simulink model "Double_track_model"  (R2025b)
settings: Solver=VariableStepAuto  StartTime=0.0  StopTime=100  MaxStep=0.001  RelTol=1e-4
model workspace (MAT data in the model file):
  A = 1
  C1 = 1.2801
  C2 = 23.99
  C3 = 0.52
  Cd = 0.01
  Croll = 0.015
  Hcg = 0.25
  Iw = 0.65
  Izz = 100
  L = 1.535
  Lf = 0.78285
  Lr = 0.75215
  M = 270
  Rw = 0.228
  b = 0.1
  rho = 1.25
  tf = 1.24
  tr = 1.24
libraries: simulink x1
settings Model: SnapshotBufferSize=1000  SnapshotInterval=1  Creator=vishal bhujbal  LastModifiedBy=vishal bhujbal
settings DebuggingCC: AlgebraicLoopMsg=none

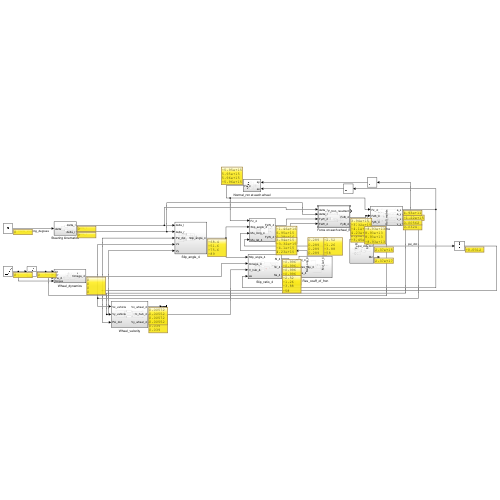
[thumbnail: Simulink's stored preview of the top-level diagram]
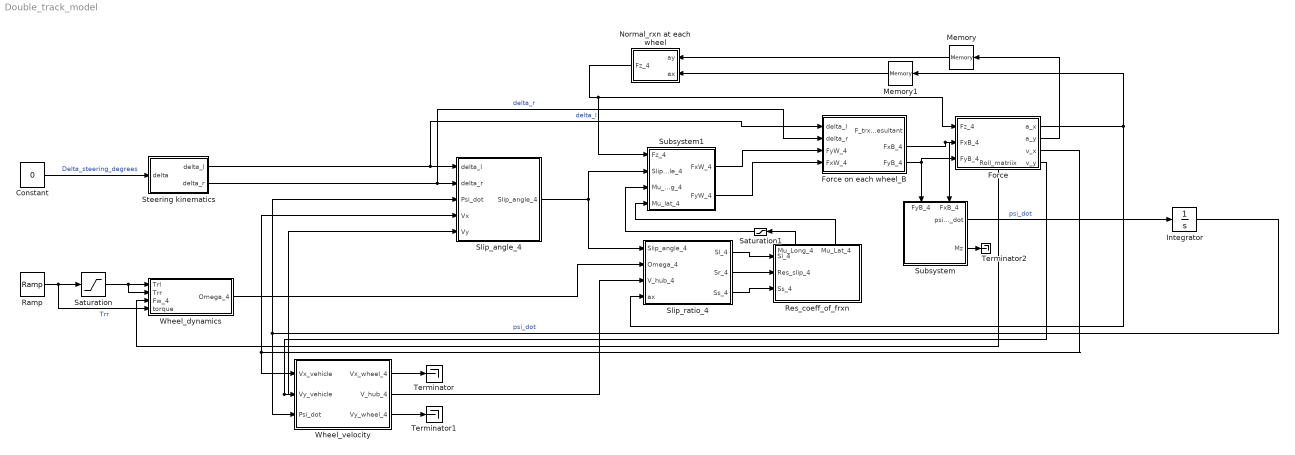
== system Double_track_model ==
  Constant : Constant  Value=0
  "Force " : Subsystem
      settings: PortSchema="{\"entries\":[{\"content\":{\"sides\":[{\"content\":{\"connectorIds\":[\"In1\",\"In2\",\"In3\"]},\"type\":\"ConnectorPlacement.EquallySpacedRectSide\",\"uuid\":\"d5a684a3-405b-4555-a50f-188f2a4da8d7\"},{\"content\":{\"connectorIds\":[\"Out1\",\"Out2\",\"Out3\",\"Out4\"],\"side\":\"RIGHT\"},\"type\":\"ConnectorPlacement.EquallySpacedRectSide\",\"uuid\":\"542d621c-7925-49ff-9525-88ce37fba4f5\"},{\"content\":{\"side\":\"TOP\"},\"type\":\"ConnectorPlacement.EquallySpacedRectSide\",\"uuid\":\"43f45826-7af5-4baa-927c-30d7ca0ba12e\"},{\"content\":{\"connectorIds\":[\"Out5\"],\"side\":\"BOTTOM\"},\"type\":\"ConnectorPlacement.EquallySpacedRectSide\",\"uuid\":\"968878bb-8701-45ce-acde-54180892fdcf\"}]},\"type\":\"ConnectorPlacement.EquallySpacedConnector\",\"uuid\":\"207dd83c-3604-4905-a41a-a8d49a457a53\"}],\"packageUris\":[\"http://schema.mathworks.com/mf0/Connector/R2020b\"],\"version\":\"1.0\"}"
  Force on each wheel_B : Subsystem
  Integrator : Integrator  InitialCondition=0.0001  ZeroCross=off
  Memory : Memory
  Memory1 : Memory
  Normal_rxn at each wheel : Subsystem
  Ramp : simulink/Sources/Ramp  slope=0  start=2  InitialOutput=0
  Res_coeff_of_frxn : Subsystem
      settings: PortSchema="{\"entries\":[{\"content\":{\"sides\":[{\"content\":{\"connectorIds\":[\"In1\",\"In2\",\"In3\"]},\"type\":\"ConnectorPlacement.EquallySpacedRectSide\",\"uuid\":\"69ce259e-3e29-48f3-954d-87ca310c7402\"},{\"content\":{\"side\":\"RIGHT\"},\"type\":\"ConnectorPlacement.EquallySpacedRectSide\",\"uuid\":\"84bf132b-ee57-474e-86e9-ab37d396531c\"},{\"content\":{\"connectorIds\":[\"Out1\",\"Out2\"],\"side\":\"TOP\"},\"type\":\"ConnectorPlacement.EquallySpacedRectSide\",\"uuid\":\"0b052469-b674-480c-8987-c0791ceb77cf\"}]},\"type\":\"ConnectorPlacement.EquallySpacedConnector\",\"uuid\":\"c5b7a706-d352-49d6-8b51-876ad1d5647c\"}],\"packageUris\":[\"http://schema.mathworks.com/mf0/Connector/R2020b\"],\"version\":\"1.0\"}"
  Saturation : Saturate  UpperLimit=29.1  LowerLimit=0
  Saturation1 : Saturate  UpperLimit=10  LowerLimit=-10
  Slip_angle_4 : Subsystem
  Slip_ratio_4 : Subsystem
  Steering kinematics : Subsystem
  Subsystem : Subsystem
      settings: PortSchema="{\"entries\":[{\"content\":{\"sides\":[{\"content\":{},\"type\":\"ConnectorPlacement.EquallySpacedRectSide\",\"uuid\":\"c1ec9233-0278-4624-8e9f-6381d2d56a9b\"},{\"content\":{\"connectorIds\":[\"Out1\",\"Out2\"],\"side\":\"RIGHT\"},\"type\":\"ConnectorPlacement.EquallySpacedRectSide\",\"uuid\":\"2db34302-ad88-4699-a49a-fe80526a01d5\"},{\"content\":{\"connectorIds\":[\"In1\",\"In2\"],\"side\":\"TOP\"},\"type\":\"ConnectorPlacement.EquallySpacedRectSide\",\"uuid\":\"531e9130-76c1-4daf-8db4-ad065a2e7511\"}]},\"type\":\"ConnectorPlacement.EquallySpacedConnector\",\"uuid\":\"470261c8-cc96-4ff8-80fc-dd2fad166e9a\"}],\"packageUris\":[\"http://schema.mathworks.com/mf0/Connector/R2020b\"],\"version\":\"1.0\"}"
  Subsystem1 : Subsystem
  Terminator : Terminator
  Terminator1 : Terminator
  Terminator2 : Terminator
  Wheel_dynamics : Subsystem
  Wheel_velocity : Subsystem
  wires:
  Steering kinematics/1(delta_l) -> Force on each wheel_B/1(delta_l), Slip_angle_4/1(delta_l)  "delta_l"
  Steering kinematics/2(delta_r) -> Force on each wheel_B/2(delta_r), Slip_angle_4/2(delta_r)  "delta_r"
  Constant/1 -> Steering kinematics/1(delta)  "Delta_steering_degrees"
  Wheel_dynamics/1(Omega_4) -> Slip_ratio_4/2(Omega_4)
  Slip_angle_4/1(Slip_angle_4) -> Subsystem1/2(Slip_angle_4), Slip_ratio_4/1(Slip_angle_4)
  Slip_ratio_4/2(Sr_4) -> Res_coeff_of_frxn/2(Res_slip_4)
  Slip_ratio_4/1(Sl_4) -> Res_coeff_of_frxn/1(Sl_4)
  Slip_ratio_4/3(Ss_4) -> Res_coeff_of_frxn/3(Ss_4)
  Normal_rxn at each wheel/1(Fz_4) -> Subsystem1/1(Fz_4), "Force "/1(Fz_4)
  Ramp/1 -> Wheel_dynamics/4(torque), Saturation/1  "Trr"
  Force on each wheel_B/2(FxB_4) -> Subsystem/2(FxB_4), "Force "/2(FxB_4)
  Force on each wheel_B/3(FyB_4) -> "Force "/3(FyB_4), Subsystem/1(FyB_4)
  "Force "/5(Roll_matriix) -> Wheel_dynamics/3(Fw_4)
  Subsystem/1(psi_dot_dot) -> Integrator/1  "psi_dot"
  Saturation/1 -> Wheel_dynamics/2(Trr), Wheel_dynamics/1(Trl)
  Wheel_velocity/3(Vy_wheel_4) -> Terminator1/1
  Wheel_velocity/1(Vx_wheel_4) -> Terminator/1
  Res_coeff_of_frxn/1(Mu_Long_4) -> Saturation1/1
  Res_coeff_of_frxn/2(Mu_Lat_4) -> Subsystem1/4(Mu_lat_4)
  Subsystem1/1(FxW_4) -> Force on each wheel_B/3(FyW_4)
  Subsystem1/2(FyW_4) -> Force on each wheel_B/4(FxW_4)
  "Force "/1(a_x) -> Memory1/1, Slip_ratio_4/4(ax)
  "Force "/2(a_y) -> Memory/1
  Subsystem/2(Mz) -> Terminator2/1
  Integrator/1 -> Wheel_velocity/3(Psi_dot), Slip_angle_4/3(Psi_dot)  "psi_dot"
  Saturation1/1 -> Subsystem1/3(Mu_long_4)
  Memory/1 -> Normal_rxn at each wheel/1(ay)
  Memory1/1 -> Normal_rxn at each wheel/2(ax)
  "Force "/3(v_x) -> Wheel_velocity/1(Vx_vehicle), Slip_angle_4/4(Vx)
  "Force "/4(v_y) -> Slip_angle_4/5(Vy), Wheel_velocity/2(Vy_vehicle)
  Wheel_velocity/2(V_hub_4) -> Slip_ratio_4/3(V_hub_4)

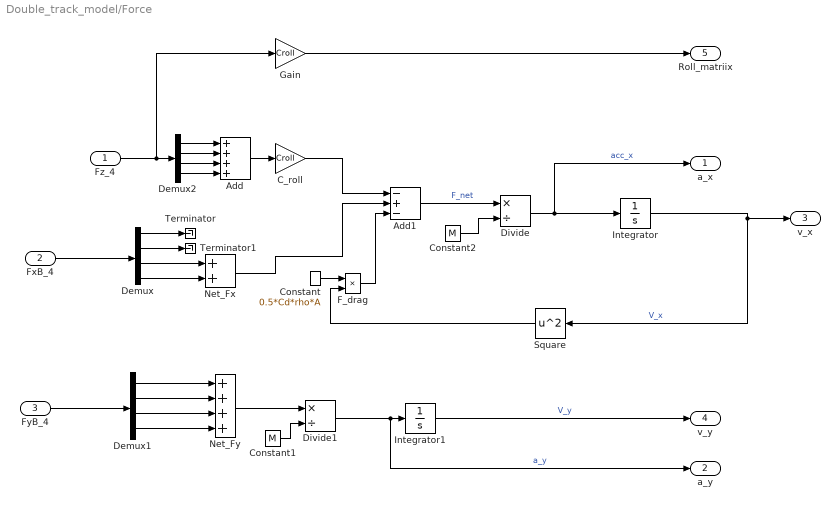
== system Double_track_model/Force  ==
  Fz_4 : Inport
  FxB_4 : Inport  Port=2
  FyB_4 : Inport  Port=3
  Add : Sum  Inputs=++++
  Add1 : Sum  Inputs=-+-
  C_roll : Gain  Gain=Croll
  Constant : Constant  Value=0.5*Cd*rho*A
  Constant1 : Constant  Value=M
  Constant2 : Constant  Value=M
  Demux : Demux
  Demux1 : Demux
  Demux2 : Demux
  Divide : Product  Inputs=*/
  Divide1 : Product  Inputs=*/
  F_drag : Product
  Gain : Gain  Gain=Croll
  Integrator : Integrator  InitialCondition=0.01
  Integrator1 : Integrator  InitialCondition=0.0001
  Net_Fx : Sum
  Net_Fy : Sum  Inputs=++++
  Square : Math  Operator=square
  Terminator : Terminator
  Terminator1 : Terminator
  a_x : Outport
  a_y : Outport  Port=2
  v_x : Outport  Port=3
  v_y : Outport  Port=4
  Roll_matriix : Outport  Port=5
  wires:
  FxB_4/1 -> Demux/1
  Demux/2 -> Terminator1/1
  Demux/1 -> Terminator/1
  Demux/3 -> Net_Fx/1
  Demux/4 -> Net_Fx/2
  FyB_4/1 -> Demux1/1
  Demux1/1 -> Net_Fy/1
  Demux1/2 -> Net_Fy/2
  Demux1/3 -> Net_Fy/3
  Demux1/4 -> Net_Fy/4
  Net_Fy/1 -> Divide1/1
  Constant1/1 -> Divide1/2
  Divide1/1 -> a_y/1, Integrator1/1  "a_y"
  Demux2/1 -> Add/1
  Demux2/2 -> Add/2
  Demux2/3 -> Add/3
  Demux2/4 -> Add/4
  Fz_4/1 -> Gain/1, Demux2/1
  Add/1 -> C_roll/1
  C_roll/1 -> Add1/1
  Net_Fx/1 -> Add1/2
  Constant/1 -> F_drag/1
  F_drag/1 -> Add1/3
  Add1/1 -> Divide/1  "F_net"
  Constant2/1 -> Divide/2
  Divide/1 -> Integrator/1, a_x/1  "acc_x"
  Integrator/1 -> v_x/1, Square/1  "V_x"
  Integrator1/1 -> v_y/1  "V_y"
  Gain/1 -> Roll_matriix/1
  Square/1 -> F_drag/2

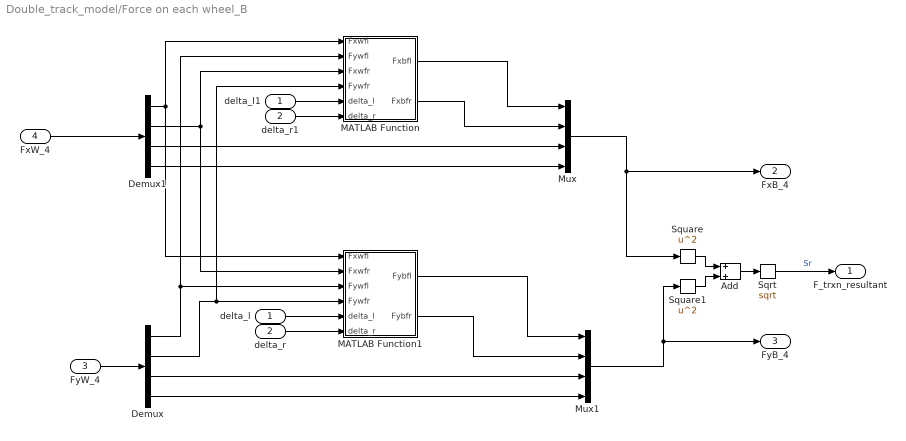
== system Double_track_model/Force on each wheel_B ==
  delta_l : Inport
  delta_r : Inport  Port=2
  FyW_4 : Inport  Port=3
  FxW_4 : Inport  Port=4
  Add : Sum
  Demux : Demux
  Demux1 : Demux
  MATLAB Function : MATLAB Function  TreatAsAtomicUnit=on
  MATLAB Function1 : MATLAB Function  TreatAsAtomicUnit=on
  Mux : Mux
  Mux1 : Mux
  Sqrt : Sqrt
  Square : Math  Operator=square
  Square1 : Math  Operator=square
  delta_l1 : InportShadow
  delta_r1 : InportShadow  Port=2
  F_trxn_resultant : Outport
  FxB_4 : Outport  Port=2
  FyB_4 : Outport  Port=3
  wires:
  FyW_4/1 -> Demux/1
  Demux1/1 -> MATLAB Function/1(Fxwfl), MATLAB Function1/1(Fxwfl)
  Demux1/2 -> MATLAB Function1/2(Fxwfr), MATLAB Function/3(Fxwfr)
  Demux1/4 -> Mux/4
  Demux1/3 -> Mux/3
  Mux/1 -> Square/1, FxB_4/1
  Demux/4 -> Mux1/4
  Demux/3 -> Mux1/3
  Demux/1 -> MATLAB Function1/3(Fywfl), MATLAB Function/2(Fywfl)
  Demux/2 -> MATLAB Function/4(Fywfr), MATLAB Function1/4(Fywfr)
  delta_r1/1 -> MATLAB Function/6(delta_r)
  delta_l1/1 -> MATLAB Function/5(delta_l)
  MATLAB Function/1(Fxbfl) -> Mux/1
  MATLAB Function/2(Fxbfr) -> Mux/2
  delta_r/1 -> MATLAB Function1/6(delta_r)
  delta_l/1 -> MATLAB Function1/5(delta_l)
  MATLAB Function1/1(Fybfl) -> Mux1/1
  MATLAB Function1/2(Fybfr) -> Mux1/2
  Mux1/1 -> Square1/1, FyB_4/1
  Square1/1 -> Add/2
  Add/1 -> Sqrt/1
  Square/1 -> Add/1
  Sqrt/1 -> F_trxn_resultant/1  "Sr"
  FxW_4/1 -> Demux1/1

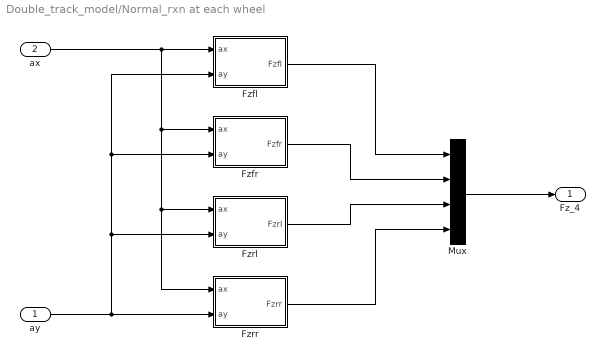
== system Double_track_model/Normal_rxn at each wheel ==
  ay : Inport
  ax : Inport  Port=2
  Fzfl : MATLAB Function  TreatAsAtomicUnit=on
  Fzfr : MATLAB Function  TreatAsAtomicUnit=on
  Fzrl : MATLAB Function  TreatAsAtomicUnit=on
  Fzrr : MATLAB Function  TreatAsAtomicUnit=on
  Mux : Mux
  Fz_4 : Outport
  wires:
  ay/1 -> Fzrl/2(ay), Fzfr/2(ay), Fzfl/2(ay), Fzrr/2(ay)
  ax/1 -> Fzfr/1(ax), Fzrl/1(ax), Fzrr/1(ax), Fzfl/1(ax)
  Fzfl/1(Fzfl) -> Mux/1
  Fzfr/1(Fzfr) -> Mux/2
  Fzrl/1(Fzrl) -> Mux/3
  Fzrr/1(Fzrr) -> Mux/4
  Mux/1 -> Fz_4/1

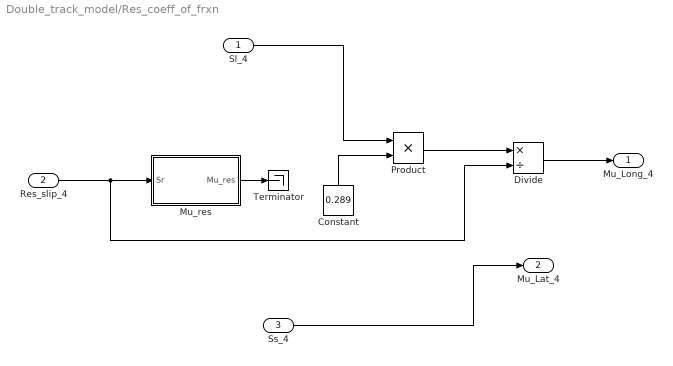
== system Double_track_model/Res_coeff_of_frxn ==
  Sl_4 : Inport
  Res_slip_4 : Inport  Port=2
  Ss_4 : Inport  Port=3
  Constant : Constant  Value=0.289
  Divide : Product  Inputs=*/
  Mu_res : MATLAB Function  TreatAsAtomicUnit=on
  Product : Product
  Terminator : Terminator
  Mu_Long_4 : Outport
  Mu_Lat_4 : Outport  Port=2
  wires:
  Constant/1 -> Product/2
  Sl_4/1 -> Product/1
  Ss_4/1 -> Mu_Lat_4/1
  Divide/1 -> Mu_Long_4/1
  Res_slip_4/1 -> Divide/2, Mu_res/1(Sr)
  Product/1 -> Divide/1
  Mu_res/1(Mu_res) -> Terminator/1

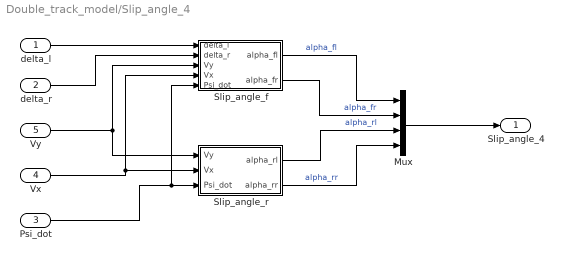
== system Double_track_model/Slip_angle_4 ==
  delta_l : Inport
  delta_r : Inport  Port=2
  Psi_dot : Inport  Port=3
  Vx : Inport  Port=4
  Vy : Inport  Port=5
  Mux : Mux
  Slip_angle_f : MATLAB Function  TreatAsAtomicUnit=on
  Slip_angle_r : MATLAB Function  TreatAsAtomicUnit=on
  Slip_angle_4 : Outport
  wires:
  delta_l/1 -> Slip_angle_f/1(delta_l)
  Vx/1 -> Slip_angle_f/4(Vx), Slip_angle_r/2(Vx)
  Psi_dot/1 -> Slip_angle_r/3(Psi_dot), Slip_angle_f/5(Psi_dot)
  Vy/1 -> Slip_angle_f/3(Vy), Slip_angle_r/1(Vy)
  delta_r/1 -> Slip_angle_f/2(delta_r)
  Slip_angle_f/1(alpha_fl) -> Mux/1  "alpha_fl"
  Slip_angle_f/2(alpha_fr) -> Mux/2  "alpha_fr"
  Slip_angle_r/1(alpha_rl) -> Mux/3  "alpha_rl"
  Slip_angle_r/2(alpha_rr) -> Mux/4  "alpha_rr"
  Mux/1 -> Slip_angle_4/1

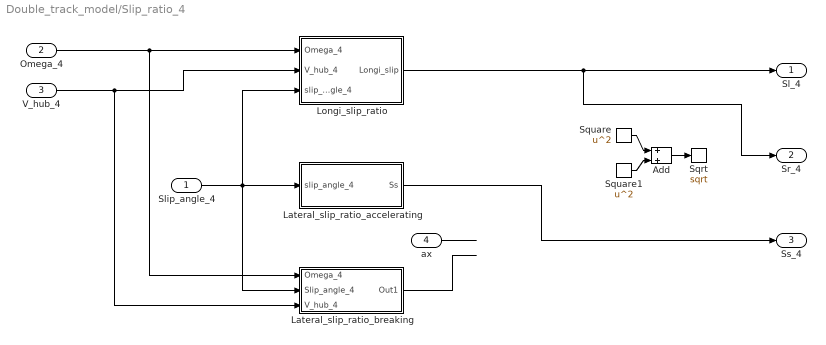
== system Double_track_model/Slip_ratio_4 ==
  Slip_angle_4 : Inport
  Omega_4 : Inport  Port=2
  V_hub_4 : Inport  Port=3
  ax : Inport  Port=4
  Add : Sum
  Lateral_slip_ratio_accelerating : Subsystem
  Lateral_slip_ratio_breaking : Subsystem
  Longi_slip_ratio : Subsystem
  Sqrt : Sqrt
  Square : Math  Operator=square
  Square1 : Math  Operator=square
  Sl_4 : Outport
  Sr_4 : Outport  Port=2
  Ss_4 : Outport  Port=3
  wires:
  Omega_4/1 -> Lateral_slip_ratio_breaking/1(Omega_4), Longi_slip_ratio/1(Omega_4)
  V_hub_4/1 -> Lateral_slip_ratio_breaking/3(V_hub_4), Longi_slip_ratio/2(V_hub_4)
  ax/1 -> ?
  Lateral_slip_ratio_accelerating/1(Ss) -> Ss_4/1
  Lateral_slip_ratio_breaking/1(Out1) -> ?
  Longi_slip_ratio/1(Longi_slip) -> Sr_4/1, Sl_4/1
  Slip_angle_4/1 -> Longi_slip_ratio/3(slip_angle_4), Lateral_slip_ratio_breaking/2(Slip_angle_4), Lateral_slip_ratio_accelerating/1(slip_angle_4)
  Square1/1 -> Add/2
  Square/1 -> Add/1
  Add/1 -> Sqrt/1

== system Double_track_model/Steering kinematics ==
  delta : Inport
  Delta_left_degrees : MATLAB Function  TreatAsAtomicUnit=on
  Delta_right_degrees : MATLAB Function  TreatAsAtomicUnit=on
  delta_l : Outport
  delta_r : Outport  Port=2
  wires:
  Delta_right_degrees/1(y) -> delta_r/1
  delta/1 -> Delta_right_degrees/1(delta), Delta_left_degrees/1(delta)
  Delta_left_degrees/1(y) -> delta_l/1

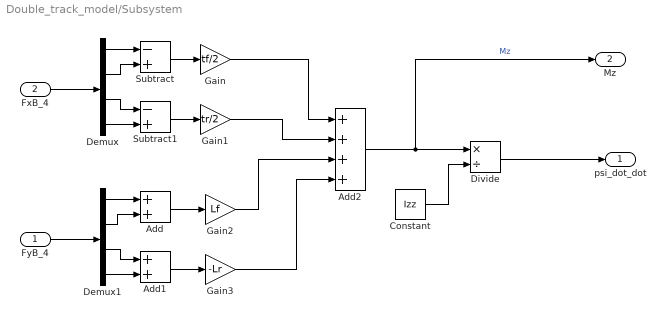
== system Double_track_model/Subsystem ==
  FyB_4 : Inport
  FxB_4 : Inport  Port=2
  Add : Sum
  Add1 : Sum
  Add2 : Sum  Inputs=++++
  Constant : Constant  Value=Izz
  Demux : Demux
  Demux1 : Demux
  Divide : Product  Inputs=*/
  Gain : Gain  Gain=tf/2
  Gain1 : Gain  Gain=tr/2
  Gain2 : Gain  Gain=Lf
  Gain3 : Gain  Gain=-Lr
  Subtract : Sum  Inputs=-+
  Subtract1 : Sum  Inputs=-+
  psi_dot_dot : Outport
  Mz : Outport  Port=2
  wires:
  FxB_4/1 -> Demux/1
  FyB_4/1 -> Demux1/1
  Demux/2 -> Subtract/2
  Demux/1 -> Subtract/1
  Subtract/1 -> Gain/1
  Gain/1 -> Add2/1
  Demux/4 -> Subtract1/2
  Demux/3 -> Subtract1/1
  Subtract1/1 -> Gain1/1
  Gain1/1 -> Add2/2
  Demux1/1 -> Add/1
  Demux1/2 -> Add/2
  Add/1 -> Gain2/1
  Demux1/3 -> Add1/1
  Demux1/4 -> Add1/2
  Add1/1 -> Gain3/1
  Gain3/1 -> Add2/4
  Gain2/1 -> Add2/3
  Add2/1 -> Mz/1, Divide/1  "Mz"
  Constant/1 -> Divide/2
  Divide/1 -> psi_dot_dot/1

== system Double_track_model/Subsystem1 ==
  Fz_4 : Inport
  Slip_angle_4 : Inport  Port=2
  Mu_long_4 : Inport  Port=3
  Mu_lat_4 : Inport  Port=4
  MATLAB Function : MATLAB Function  TreatAsAtomicUnit=on
  FxW_4 : Outport
  FyW_4 : Outport  Port=2
  wires:
  MATLAB Function/1(FxW_4) -> FxW_4/1
  MATLAB Function/2(FyW_4) -> FyW_4/1
  Fz_4/1 -> MATLAB Function/4(Fz_4)
  Mu_lat_4/1 -> MATLAB Function/3(Mu_lat_4)
  Mu_long_4/1 -> MATLAB Function/2(Mu_long_4)
  Slip_angle_4/1 -> MATLAB Function/1(slip_angle_4)

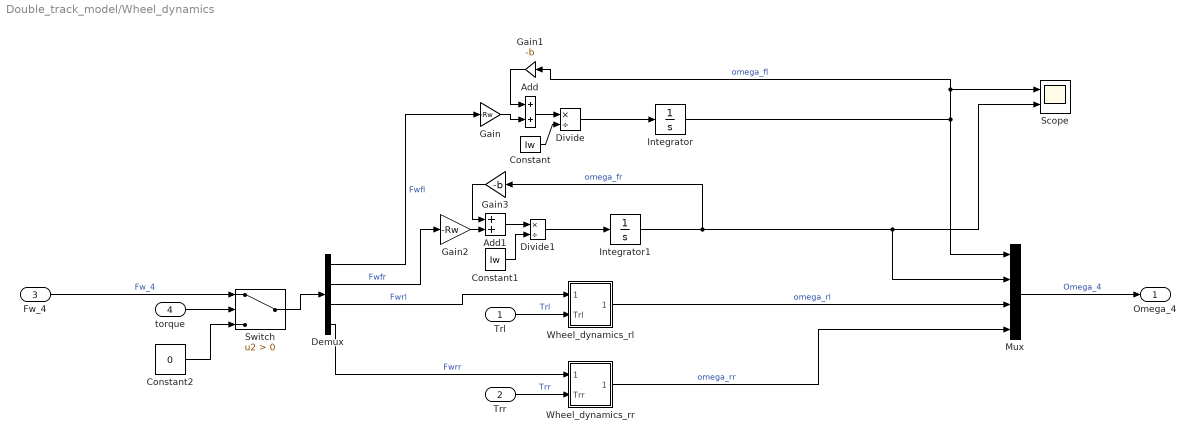
== system Double_track_model/Wheel_dynamics ==
  Trl : Inport
  Trr : Inport  Port=2
  Fw_4 : Inport  Port=3
  torque : Inport  Port=4
  Add : Sum
  Add1 : Sum
  Constant : Constant  Value=Iw
  Constant1 : Constant  Value=Iw
  Constant2 : Constant  Value=0
  Demux : Demux
  Divide : Product  Inputs=*/
  Divide1 : Product  Inputs=*/
  Gain : Gain  Gain=-Rw
  Gain1 : Gain  Gain=-b
  Gain2 : Gain  Gain=-Rw
  Gain3 : Gain  Gain=-b
  Integrator : Integrator
  Integrator1 : Integrator
  Mux : Mux
  Scope : Scope  NumInputPorts=2
  Switch : Switch  Criteria=u2 > Threshold  SaturateOnIntegerOverflow=off  InputSameDT=off
  Wheel_dynamics_rl : Subsystem
  Wheel_dynamics_rr : Subsystem
  Omega_4 : Outport
  wires:
  Trl/1 -> Wheel_dynamics_rl/2(Trl)  "Trl"
  Trr/1 -> Wheel_dynamics_rr/2(Trr)  "Trr"
  Fw_4/1 -> Switch/1  "Fw_4"
  Demux/1 -> Gain/1  "Fwfl"
  Demux/2 -> Gain2/1  "Fwfr"
  Demux/3 -> Wheel_dynamics_rl/1(Fwrl)  "Fwrl"
  Demux/4 -> Wheel_dynamics_rr/1(Fwrr)  "Fwrr"
  Wheel_dynamics_rl/1(Out1) -> Mux/3  "omega_rl"
  Wheel_dynamics_rr/1(Out1) -> Mux/4  "omega_rr"
  Mux/1 -> Omega_4/1  "Omega_4"
  Divide/1 -> Integrator/1
  Integrator1/1 -> Gain3/1, Scope/2, Mux/2  "omega_fr"
  Gain/1 -> Add/2
  Add/1 -> Divide/1
  Gain1/1 -> Add/1
  Constant/1 -> Divide/2
  Add1/1 -> Divide1/1
  Gain2/1 -> Add1/2
  Constant1/1 -> Divide1/2
  Gain3/1 -> Add1/1
  Divide1/1 -> Integrator1/1
  Integrator/1 -> Mux/1, Gain1/1, Scope/1  "omega_fl"
  torque/1 -> Switch/2
  Constant2/1 -> Switch/3
  Switch/1 -> Demux/1

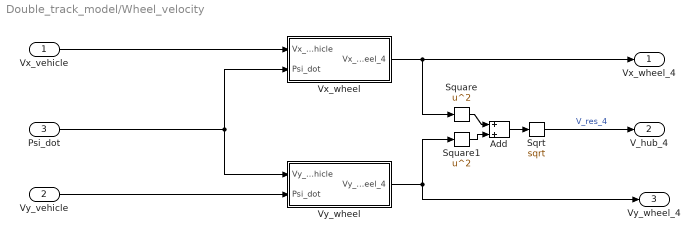
== system Double_track_model/Wheel_velocity ==
  Vx_vehicle : Inport
  Vy_vehicle : Inport  Port=2
  Psi_dot : Inport  Port=3
  Add : Sum
  Sqrt : Sqrt
  Square : Math  Operator=square
  Square1 : Math  Operator=square
  Vx_wheel : Subsystem
  Vy_wheel : Subsystem
  Vx_wheel_4 : Outport
  V_hub_4 : Outport  Port=2
  Vy_wheel_4 : Outport  Port=3
  wires:
  Vx_wheel/1(Vx_wheel_4) -> Square/1, Vx_wheel_4/1
  Vy_wheel/1(Vy_wheel_4) -> Square1/1, Vy_wheel_4/1
  Sqrt/1 -> V_hub_4/1  "V_res_4"
  Psi_dot/1 -> Vy_wheel/1(Vy_vehicle), Vx_wheel/2(Psi_dot)
  Vx_vehicle/1 -> Vx_wheel/1(Vx_vehicle)
  Vy_vehicle/1 -> Vy_wheel/2(Psi_dot)
  Square/1 -> Add/1
  Square1/1 -> Add/2
  Add/1 -> Sqrt/1

== system Double_track_model/Slip_ratio_4/Lateral_slip_ratio_accelerating ==
  slip_angle_4 : Inport
  MATLAB Function : MATLAB Function  TreatAsAtomicUnit=on
  Ss : Outport
  wires:
  slip_angle_4/1 -> MATLAB Function/1(slip_angle_4)
  MATLAB Function/1(Ss) -> Ss/1

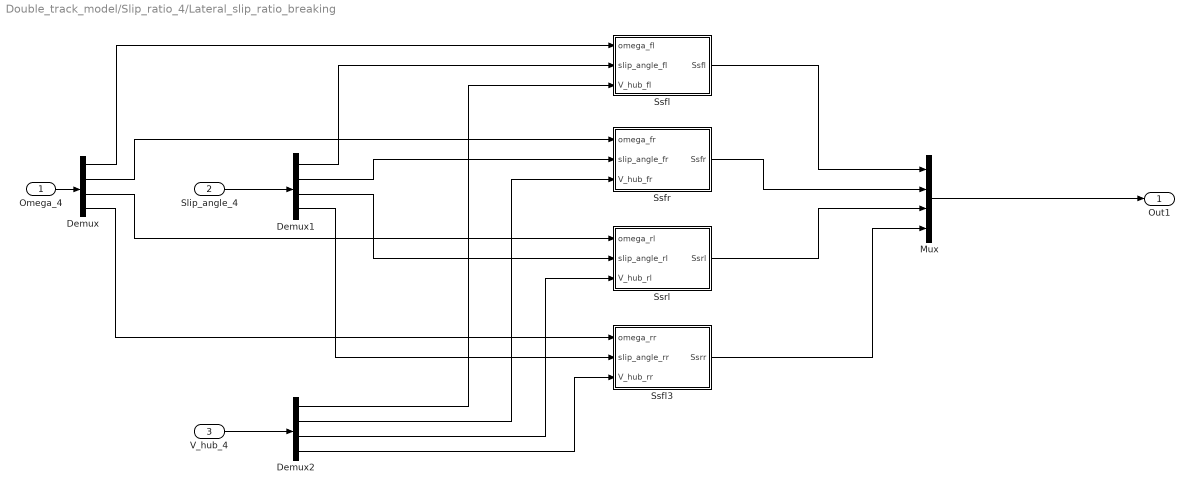
== system Double_track_model/Slip_ratio_4/Lateral_slip_ratio_breaking ==
  Omega_4 : Inport
  Slip_angle_4 : Inport  Port=2
  V_hub_4 : Inport  Port=3
  Demux : Demux
  Demux1 : Demux
  Demux2 : Demux
  Mux : Mux
  Ssfl : MATLAB Function  TreatAsAtomicUnit=on
  Ssfl3 : MATLAB Function  TreatAsAtomicUnit=on
  Ssfr : MATLAB Function  TreatAsAtomicUnit=on
  Ssrl : MATLAB Function  TreatAsAtomicUnit=on
  Out1 : Outport
  wires:
  Omega_4/1 -> Demux/1
  Demux/1 -> Ssfl/1(omega_fl)
  Demux/4 -> Ssfl3/1(omega_rr)
  Demux/2 -> Ssfr/1(omega_fr)
  Demux/3 -> Ssrl/1(omega_rl)
  Slip_angle_4/1 -> Demux1/1
  Demux1/1 -> Ssfl/2(slip_angle_fl)
  Demux1/2 -> Ssfr/2(slip_angle_fr)
  Demux1/3 -> Ssrl/2(slip_angle_rl)
  Demux1/4 -> Ssfl3/2(slip_angle_rr)
  V_hub_4/1 -> Demux2/1
  Demux2/1 -> Ssfl/3(V_hub_fl)
  Demux2/2 -> Ssfr/3(V_hub_fr)
  Demux2/3 -> Ssrl/3(V_hub_rl)
  Demux2/4 -> Ssfl3/3(V_hub_rr)
  Ssfl/1(Ssfl) -> Mux/1
  Ssfr/1(Ssfr) -> Mux/2
  Ssrl/1(Ssrl) -> Mux/3
  Ssfl3/1(Ssrr) -> Mux/4
  Mux/1 -> Out1/1

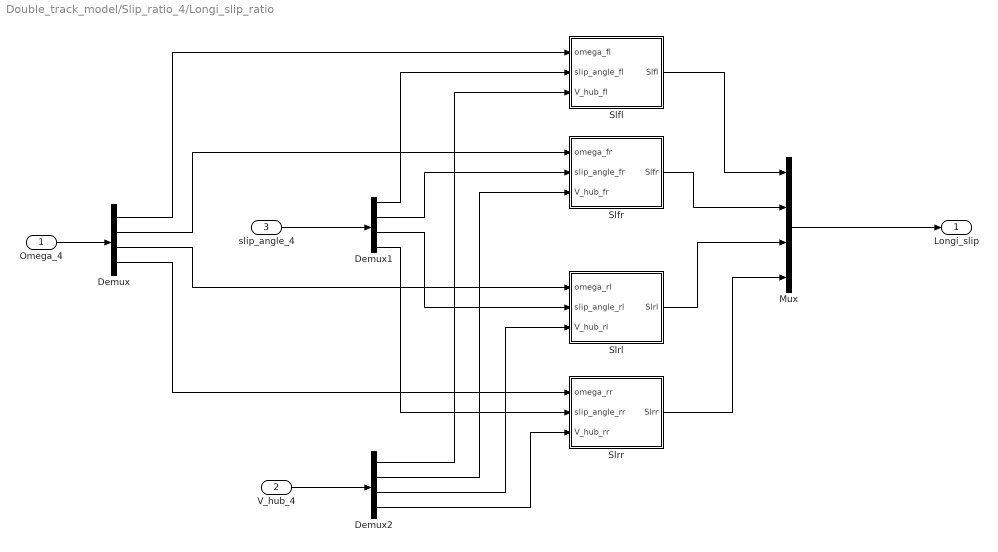
== system Double_track_model/Slip_ratio_4/Longi_slip_ratio ==
  Omega_4 : Inport
  V_hub_4 : Inport  Port=2
  slip_angle_4 : Inport  Port=3
  Demux : Demux
  Demux1 : Demux
  Demux2 : Demux
  Mux : Mux
  Slfl : MATLAB Function  TreatAsAtomicUnit=on
  Slfr : MATLAB Function  TreatAsAtomicUnit=on
  Slrl : MATLAB Function  TreatAsAtomicUnit=on
  Slrr : MATLAB Function  TreatAsAtomicUnit=on
  Longi_slip : Outport
  wires:
  Omega_4/1 -> Demux/1
  Demux/1 -> Slfl/1(omega_fl)
  Demux/2 -> Slfr/1(omega_fr)
  Demux/3 -> Slrl/1(omega_rl)
  Demux/4 -> Slrr/1(omega_rr)
  Demux1/1 -> Slfl/2(slip_angle_fl)
  Demux1/2 -> Slfr/2(slip_angle_fr)
  Demux1/3 -> Slrl/2(slip_angle_rl)
  Demux1/4 -> Slrr/2(slip_angle_rr)
  slip_angle_4/1 -> Demux1/1
  V_hub_4/1 -> Demux2/1
  Demux2/1 -> Slfl/3(V_hub_fl)
  Demux2/2 -> Slfr/3(V_hub_fr)
  Demux2/3 -> Slrl/3(V_hub_rl)
  Demux2/4 -> Slrr/3(V_hub_rr)
  Slfl/1(Slfl) -> Mux/1
  Slfr/1(Slfr) -> Mux/2
  Slrl/1(Slrl) -> Mux/3
  Slrr/1(Slrr) -> Mux/4
  Mux/1 -> Longi_slip/1

== system Double_track_model/Wheel_dynamics/Wheel_dynamics_rl ==
  Fwrl : Inport
  Trl : Inport  Port=2
  Integrator : Integrator
  MATLAB Function : MATLAB Function  TreatAsAtomicUnit=on
  Out1 : Outport
  wires:
  MATLAB Function/1(omega_dot_rl) -> Integrator/1  "w_dot"
  Integrator/1 -> Out1/1, MATLAB Function/3(omega_rl)  "Omega_rl"
  Fwrl/1 -> MATLAB Function/2(Fwrl)
  Trl/1 -> MATLAB Function/1(Trl)

== system Double_track_model/Wheel_dynamics/Wheel_dynamics_rr ==
  Fwrr : Inport
  Trr : Inport  Port=2
  Integrator : Integrator
  MATLAB Function : MATLAB Function  TreatAsAtomicUnit=on
  Out1 : Outport
  wires:
  Trr/1 -> MATLAB Function/1(Trr)
  Fwrr/1 -> MATLAB Function/2(Fwrr)
  Integrator/1 -> MATLAB Function/3(omega_rr), Out1/1  "Omega_rr"
  MATLAB Function/1(omega_dot_rr) -> Integrator/1  "w_dot"

== system Double_track_model/Wheel_velocity/Vx_wheel ==
  Vx_vehicle : Inport
  Psi_dot : Inport  Port=2
  MATLAB Function : MATLAB Function  TreatAsAtomicUnit=on
  Mux : Mux
  Vx_wheel_4 : Outport
  wires:
  Vx_vehicle/1 -> MATLAB Function/1(Vx_vehicle)
  Psi_dot/1 -> MATLAB Function/2(Psi_dot)
  MATLAB Function/1(Vxwfl) -> Mux/1
  MATLAB Function/2(Vxwfr) -> Mux/2
  MATLAB Function/3(Vxwrl) -> Mux/3
  MATLAB Function/4(Vxwrr) -> Mux/4
  Mux/1 -> Vx_wheel_4/1

== system Double_track_model/Wheel_velocity/Vy_wheel ==
  Vy_vehicle : Inport
  Psi_dot : Inport  Port=2
  MATLAB Function : MATLAB Function  TreatAsAtomicUnit=on
  Mux : Mux
  Vy_wheel_4 : Outport
  wires:
  Mux/1 -> Vy_wheel_4/1
  MATLAB Function/4(Vywrr) -> Mux/4
  MATLAB Function/3(Vywrl) -> Mux/3
  MATLAB Function/2(Vywfr) -> Mux/2
  MATLAB Function/1(Vywfl) -> Mux/1
  Psi_dot/1 -> MATLAB Function/2(Psi_dot)
  Vy_vehicle/1 -> MATLAB Function/1(Vy_vehicle)

== matlab function Double_track_model/Slip_ratio_4/Longi_slip_ratio/Slfr ==
  data: omega_fr input; Slfr output; slip_angle_fr input; V_hub_fr input
function Slfr = fcn(omega_fr,slip_angle_fr,V_hub_fr)
Rw = 0.228;
% numerator
num = omega_fr * Rw * cosd(slip_angle_fr) - V_hub_fr;

% raw denominator
den_raw = max(V_hub_fr, omega_fr * Rw * cosd(slip_angle_fr));

% create safe denominator:
% - keep the sign
% - avoid zero
% - smooth for solver
den = den_raw + sign(den_raw) * 0.0001;

% if the raw denominator is exactly zero → choose a tiny positive number
if den_raw == 0
    den = 0.0001;
end

% slip ratio
Slfr = num / den;

== matlab function Double_track_model/Slip_ratio_4/Longi_slip_ratio/Slrl ==
  data: omega_rl input; Slrl output; slip_angle_rl input; V_hub_rl input
function Slrl = fcn(omega_rl,slip_angle_rl,V_hub_rl)
Rw = 0.228;
% numerator
num = omega_rl * Rw * cosd(slip_angle_rl) - V_hub_rl;

% raw denominator
den_raw = max(V_hub_rl, omega_rl * Rw * cosd(slip_angle_rl));

% create safe denominator:
% - keep the sign
% - avoid zero
% - smooth for solver
den = den_raw + sign(den_raw) * 0.0001;

% if the raw denominator is exactly zero → choose a tiny positive number
if den_raw == 0
    den = 0.0001;
end

% slip ratio
Slrl = num / den;

== matlab function Double_track_model/Slip_ratio_4/Longi_slip_ratio/Slrr ==
  data: omega_rr input; Slrr output; slip_angle_rr input; V_hub_rr input
function Slrr = fcn(omega_rr, slip_angle_rr, V_hub_rr)
Rw = 0.228;
% numerator
num = omega_rr * Rw * cosd(slip_angle_rr) - V_hub_rr;

% raw denominator
den_raw = max(V_hub_rr, omega_rr * Rw * cosd(slip_angle_rr));

% create safe denominator:
% - keep the sign
% - avoid zero
% - smooth for solver
den = den_raw + sign(den_raw) * 0.0001;

% if the raw denominator is exactly zero → choose a tiny positive number
if den_raw == 0
    den = 0.0001;
end

% slip ratio
Slrr = num / den;

== matlab function Double_track_model/Slip_ratio_4/Longi_slip_ratio/Slfl ==
  data: omega_fl input; Slfl output; slip_angle_fl input; V_hub_fl input
function Slfl = fcn(omega_fl,slip_angle_fl,V_hub_fl)
Rw = 0.228;
% numerator
num = omega_fl * Rw * cosd(slip_angle_fl) - V_hub_fl;

% raw denominator
den_raw = max(V_hub_fl, omega_fl * Rw * cosd(slip_angle_fl));

% create safe denominator:
% - keep the sign
% - avoid zero
% - smooth for solver
den = den_raw + sign(den_raw) * 0.0001;

% if the raw denominator is exactly zero → choose a tiny positive number
if den_raw == 0
    den = 0.0001;
end

% slip ratio
Slfl = num / den;

== matlab function Double_track_model/Slip_ratio_4/Lateral_slip_ratio_breaking/Ssfl ==
  data: omega_fl input; Ssfl output; slip_angle_fl input; V_hub_fl input
function Ssfl = fcn(omega_fl,slip_angle_fl,V_hub_fl)
Rw = 0.228;
% numerator
num = omega_fl * Rw * sind(slip_angle_fl);

% raw denominator
den_raw = V_hub_fl;

% create safe denominator:
% - keep the sign
% - avoid zero
% - smooth for solver
den = den_raw + sign(den_raw) * 0.001;

% if the raw denominator is exactly zero → choose a tiny positive number
if den_raw == 0
    den = 0.001;
end

% lateral slip
Ssfl = num / den;

== matlab function Double_track_model/Slip_ratio_4/Lateral_slip_ratio_breaking/Ssfr ==
  data: omega_fr input; Ssfr output; slip_angle_fr input; V_hub_fr input
function Ssfr = fcn(omega_fr,slip_angle_fr,V_hub_fr)
Rw = 0.228;
% numerator
num = omega_fr * Rw * sind(slip_angle_fr);

% raw denominator
den_raw = V_hub_fr;

% create safe denominator:
% - keep the sign
% - avoid zero
% - smooth for solver
den = den_raw + sign(den_raw) * 0.001;

% if the raw denominator is exactly zero → choose a tiny positive number
if den_raw == 0
    den = 0.001;
end

% lateral slip
Ssfr = num / den;

== matlab function Double_track_model/Steering kinematics/Delta_right_degrees ==
  data: delta input; y output
function y = fcn(delta)
L = 1.535;
tf = 1.24;
y = atand(L/(L.*cotd(delta)+tf/2));

== matlab function Double_track_model/Slip_ratio_4/Lateral_slip_ratio_breaking/Ssrl ==
  data: omega_rl input; Ssrl output; slip_angle_rl input; V_hub_rl input
function Ssrl = fcn(omega_rl,slip_angle_rl,V_hub_rl)
Rw = 0.228;
% numerator
num = omega_rl * Rw * sind(slip_angle_rl);

% raw denominator
den_raw = V_hub_rl;

% create safe denominator:
% - keep the sign
% - avoid zero
% - smooth for solver
den = den_raw + sign(den_raw) * 0.001;

% if the raw denominator is exactly zero → choose a tiny positive number
if den_raw == 0
    den = 0.001;
end

% lateral slip
Ssrl = num / den;

== matlab function Double_track_model/Slip_ratio_4/Lateral_slip_ratio_breaking/Ssfl3 ==
  data: omega_rr input; Ssrr output; slip_angle_rr input; V_hub_rr input
function Ssrr = fcn(omega_rr,slip_angle_rr,V_hub_rr)
Rw = 0.228;
% numerator
num = omega_rr * Rw * sind(slip_angle_rr);

% raw denominator
den_raw = V_hub_rr;

% create safe denominator:
% - keep the sign
% - avoid zero
% - smooth for solver
den = den_raw + sign(den_raw) * 0.001;

% if the raw denominator is exactly zero → choose a tiny positive number
if den_raw == 0
    den = 0.001;
end

% lateral slip
Ssrr = num / den;

== matlab function Double_track_model/Slip_ratio_4/Lateral_slip_ratio_accelerating/MATLAB Function ==
  data: slip_angle_4 input; Ss output
function Ss = fcn(slip_angle_4)

Ss = tand(slip_angle_4);

== matlab function Double_track_model/Normal_rxn at each wheel/Fzfl ==
  data: ax input; Fzfl output; ay input
function Fzfl = fcn(ax,ay)

tf = 1.24;
Lf = 1.535*0.51;
L = 1.535;
Hcg = 0.25;
M = 270;

Fzfl = M*(Lf*9.81/L - Hcg.*ax/L)*(1/2-Hcg.*ay/(tf*9.81));

== matlab function Double_track_model/Normal_rxn at each wheel/Fzfr ==
  data: ax input; Fzfr output; ay input
function Fzfr = fcn(ax,ay)

tf = 1.24;
Lf = 1.535*0.51;
L = 1.535;
Hcg = 0.25;
M = 270;

Fzfr = M*(Lf*9.81/L - Hcg.*ax/L)*(1/2+Hcg.*ay/(tf*9.81));

== matlab function Double_track_model/Normal_rxn at each wheel/Fzrl ==
  data: ax input; Fzrl output; ay input
function Fzrl = fcn(ax,ay)

tr = 1.24;
Lr = 1.535*0.51;
L = 1.535;
Hcg = 0.25;
M = 270;
Fzrl = M*(Lr*9.81/L + Hcg.*ax/L)*(1/2-Hcg.*ay/(tr*9.81));

== matlab function Double_track_model/Normal_rxn at each wheel/Fzrr ==
  data: ax input; Fzrr output; ay input
function Fzrr = fcn(ax,ay)

tr = 1.24;
Lr = 1.535*0.51;
L = 1.535;
Hcg = 0.25;
M = 270;
Fzrr = M*(Lr*9.81/L + Hcg.*ax/L)*(1/2+Hcg.*ay/(tr*9.81));

== matlab function Double_track_model/Res_coeff_of_frxn/Mu_res ==
  data: Sr input; Mu_res output
function Mu_res = fcn(Sr)

C1 = 1.2801;
C2 = 23.99;
C3 = 0.52;

Mu_res = C1*(1 - exp(-C2*Sr)) - C3*Sr ;

== matlab function Double_track_model/Steering kinematics/Delta_left_degrees ==
  data: delta input; y output
function y = fcn(delta)
L = 1.535;
tf = 1.24;
y = atand(L/(L.*cotd(delta)-tf/2));

== matlab function Double_track_model/Force on each wheel_B/MATLAB Function ==
  data: Fxwfl input; Fxbfl output; Fywfl input; Fxwfr input; Fywfr input; delta_l input; delta_r input; Fxbfr output
function [Fxbfl,Fxbfr] = fcn(Fxwfl,Fywfl,Fxwfr,Fywfr,delta_l,delta_r)

Fxbfl = Fxwfl.*cosd(delta_l)-Fywfl.*sind(delta_l);

Fxbfr = Fxwfr.*cosd(delta_r)-Fywfr.*sind(delta_r);

== matlab function Double_track_model/Force on each wheel_B/MATLAB Function1 ==
  data: Fybfl output; Fxwfl input; Fxwfr input; Fywfl input; Fywfr input; delta_l input; delta_r input; Fybfr output
function [Fybfl,Fybfr] = fcn(Fxwfl,Fxwfr,Fywfl,Fywfr,delta_l,delta_r)

Fybfl = Fywfl.*cosd(delta_l)+Fxwfl.*sind(delta_l);

Fybfr = Fywfr.*cosd(delta_r)+ Fxwfr.*sind(delta_r);

== matlab function Double_track_model/Wheel_dynamics/Wheel_dynamics_rl/MATLAB Function ==
  data: Trl input; Fwrl input; omega_dot_rl output; omega_rl input
function omega_dot_rl = fcn(Trl,Fwrl,omega_rl)

Rw = 0.228;
b = 0.01;

omega_dot_rl = Trl-Fwrl.*Rw-b.*omega_rl ;

== matlab function Double_track_model/Wheel_dynamics/Wheel_dynamics_rr/MATLAB Function ==
  data: Trr input; Fwrr input; omega_dot_rr output; omega_rr input
function omega_dot_rr = fcn(Trr,Fwrr,omega_rr)

Rw = 0.228;
b = 0.01;

omega_dot_rr = Trr-Fwrr.*Rw-b.*omega_rr ;

== matlab function Double_track_model/Slip_angle_4/Slip_angle_f ==
  data: delta_l input; delta_r input; alpha_fl output; Vy input; Vx input; Psi_dot input; alpha_fr output
function [alpha_fl,alpha_fr]= fcn(delta_l,delta_r,Vy,Vx,Psi_dot)

Rw = 0.228;
tf = 1.24;
Lf = 1.535*0.51;

alpha_fl = delta_l- atand((Vy+Psi_dot.*Rw.*cosd(atand(tf/(2*Lf)).*Rw))/(Vx-Psi_dot.*Rw.*sind(atand(tf/(2*Lf))))) ;

alpha_fr = delta_r- atand((Vy+Psi_dot.*cosd(atand(tf/(2*Lf)).*Rw))/(Vx+Psi_dot.*Rw.*sind(atand(tf/(2*Lf))))) ;

== matlab function Double_track_model/Slip_angle_4/Slip_angle_r ==
  data: alpha_rl output; Vy input; Vx input; Psi_dot input; alpha_rr output
function [alpha_rl,alpha_rr]= fcn(Vy,Vx,Psi_dot)

Rw = 0.228;
tr = 1.24;
Lr = 1.535*0.49;

alpha_rl = -atand((Vy-Psi_dot.*Rw.*cosd(atand(tr/(2*Lr)).*Rw))/(Vx-Psi_dot.*Rw*sind(atand(tr/(2*Lr))))) ;

alpha_rr = -atand((Vy-Psi_dot.*cosd(atand(tr/(2*Lr)).*Rw))/(Vx+Psi_dot.*Rw.*sind(atand(tr/(2*Lr))))) ;

== matlab function Double_track_model/Subsystem1/MATLAB Function ==
  data: slip_angle_4 input; Mu_long_4 input; Mu_lat_4 input; Fz_4 input; FxW_4 output; FyW_4 output
function [FxW_4,FyW_4] = fcn(slip_angle_4,Mu_long_4,Mu_lat_4,Fz_4)

FxW_4 = Mu_long_4.*Fz_4.*cosd(slip_angle_4) + Mu_lat_4.*Fz_4.*sind(slip_angle_4);
FyW_4 = Mu_lat_4.*Fz_4.*cosd(slip_angle_4) - Mu_long_4.*Fz_4.*sind(slip_angle_4);

== matlab function Double_track_model/Wheel_velocity/Vx_wheel/MATLAB Function ==
  data: Vx_vehicle input; Vxwfl output; Psi_dot input; Vxwfr output; Vxwrl output; Vxwrr output
function [Vxwfl,Vxwfr,Vxwrl,Vxwrr] = fcn(Vx_vehicle,Psi_dot)

Rw = 0.228;
tf = 1.24;
tr = 1.24;
Lf = 1.535*0.51;
Lr = 1.535*0.49;

Vxwfl = Vx_vehicle - Psi_dot.*Rw.*sind(tf/(2.*Lf));
Vxwfr = Vx_vehicle + Psi_dot.*Rw.*sind(tf/(2.*Lf));
Vxwrl = Vx_vehicle - Psi_dot.*Rw.*sind(tr/(2.*Lr));
Vxwrr = Vx_vehicle + Psi_dot.*Rw.*sind(tr/(2.*Lr));

== matlab function Double_track_model/Wheel_velocity/Vy_wheel/MATLAB Function ==
  data: Vy_vehicle input; Vywfl output; Psi_dot input; Vywfr output; Vywrl output; Vywrr output
function [Vywfl,Vywfr,Vywrl,Vywrr] = fcn(Vy_vehicle,Psi_dot)

Rw = 0.228;
tf = 1.24;
tr = 1.24;
Lf = 1.535*0.51;
Lr = 1.535*0.49;

Vywfl = Vy_vehicle + Psi_dot.*Rw.*cosd(tf/(2.*Lf));
Vywfr = Vy_vehicle + Psi_dot.*Rw.*cosd(tf/(2.*Lf));
Vywrl = Vy_vehicle - Psi_dot.*Rw.*cosd(tr/(2.*Lr));
Vywrr = Vy_vehicle - Psi_dot.*Rw.*cosd(tr/(2.*Lr));
